simulink model "leg_contral_from_joy"  (R2024a)
settings: Solver=FixedStepDiscrete  StartTime=0.0  StopTime=inf  FixedStep=0.01  RelTol=1e-3  EnableMultiTasking=on
InitFcn:
  | run('robota_init.m')
values from neighbouring files (symbols this model uses):
  foot_step_x = single([0.647962241881123,0.669281948440417,0.689047458853030,0.707336632089232,0.724214871275340,0.739734081466605,0.753932398834638,0.766834545548556,0.778452679930586,0.788787625824203,0.797830378556315,0.805563797434742,0.811964406427908,0.817004235554845,0.820652645599333,0.822878088081130,0.823649760998204,0.822939128724922,0.820721281639968,0.816976117592065,0.811689333218330,0.804853218436 ...(+3308 chars)    [robota_init.m]
  foot_step_y = single([0.00431677655718721,0.0162618273816606,0.0344599539851875,0.0576998848000865,0.0849190036162384,0.115189239656799,0.147704049746776,0.181766425758056,0.216777863221598,0.252228229678260,0.287686473989677,0.322792120445942,0.357247494083859,0.390810626164481,0.423288791248474,0.454532629749211,0.484430812233581,0.512905204076631,0.539906491355785,0.565410231091200,0.589413291098898,0.611930 ...(+3410 chars)    [robota_init.m]
  height_plane = 0.025    [robota_init.m]
undefined symbols (not defined in the file or in its folder): axes, axes_SL_Info, buttons, buttons_SL_Info, foot_z, header, lb_alfa, lb_beta, lb_gamma, lf_alfa, lf_beta, lf_gamma, plane_x, plane_y, rb_alfa, rb_beta, rb_gamma, rf_alfa, rf_beta, rf_gamma, x, X, y, Y, z, Z
libraries: sm_lib x84, nesl_utility x21, hdlsllib x20, ros2lib x10, instrumentseriallib x2
(part 3 of 3)

== system leg_contral_from_joy/mutibody_sim/RB_Subsystem/L_jiont1 ==
  L_jiont : sm_lib/Body Elements/File Solid  ExtGeomFileName=STL/L_arm_joint.stl  UnitType=Custom  ExtGeomFileUnits=mm  StepReaderType=HEX  ExportConvexHullGeometry=off  InertiaType=Custom  BasedOnType=Density  Density=1000  DensityUnits=kg/m^3  Mass=100  MassUnits=g  CenterOfMass=[0 0 0]  CenterOfMassUnits=m  MomentsOfInertia=[1 1 1]  MomentsOfInertiaUnits=kg*m^2  ProductsOfInertia=[0 0 0]  ProductsOfInertiaUnits=kg*m^2  GraphicType=FromGeometry  MarkerShape=Sphere  MarkerSize=10  GraphicVisPropType=SimpleVisualProperties  GraphicDiffuseColor=[0.5 0.5 0.5]  GraphicOpacity=1.0  GraphicSpecularColor=[0.5 0.5 0.5 1.0]  GraphicAmbientColor=[0.15 0.15 0.15 1.0]  GraphicEmissiveColor=[0.0 0.0 0.0 1.0]  GraphicShininess=75  DoExposeReferenceFrame=on  SerializedFrames=<Frames/>
  L_jiont to Body : sm_lib/Frames and Transforms/Rigid Transform  RotationMethod=None  FollAlignAxisA=+Z  BaseAlignAxisA=+X  FollAlignAxisB=+Y  BaseAlignAxisB=+Z  RotationStandardAxis=+X  RotationAngle=180  RotationAngleUnits=deg  RotationArbitraryAxis=[0 0 1]  RotationSequenceAxes=FollowerAxes  RotationSequence=XYX  RotationSequenceAngles=[0 0 0]  RotationSequenceAnglesUnits=deg  RotationMatrix=[1 0 0; 0 1 0; 0 0 1]  Quaternion=[1 0 0 0]  TranslationMethod=Cartesian  TranslationCartesianOffset=[10 -13 9.5]  TranslationCartesianOffsetUnits=mm  TranslationStandardAxis=+Z  TranslationStandardOffset=100  TranslationStandardOffsetUnits=mm  TranslationROffset=0  TranslationROffsetUnits=m  TranslationThetaOffset=0  TranslationThetaOffsetUnits=deg  TranslationZOffset=0  TranslationZOffsetUnits=m
  L_jiont to Body1 : sm_lib/Frames and Transforms/Rigid Transform  RotationMethod=StandardAxis  FollAlignAxisA=+Z  BaseAlignAxisA=-Y  FollAlignAxisB=+Y  BaseAlignAxisB=+Z  RotationStandardAxis=+X  RotationAngle=90  RotationAngleUnits=deg  RotationArbitraryAxis=[0 0 1]  RotationSequenceAxes=FollowerAxes  RotationSequence=XYX  RotationSequenceAngles=[0 0 0]  RotationSequenceAnglesUnits=deg  RotationMatrix=[1 0 0; 0 1 0; 0 0 1]  Quaternion=[1 0 0 0]  TranslationMethod=None  TranslationCartesianOffset=[10 -13 0]  TranslationCartesianOffsetUnits=cm  TranslationStandardAxis=+Z  TranslationStandardOffset=100  TranslationStandardOffsetUnits=cm  TranslationROffset=0  TranslationROffsetUnits=m  TranslationThetaOffset=0  TranslationThetaOffsetUnits=deg  TranslationZOffset=0  TranslationZOffsetUnits=m
  "L_jiont to L_arm_ly " : sm_lib/Frames and Transforms/Rigid Transform  RotationMethod=AlignedAxes  FollAlignAxisA=+Z  BaseAlignAxisA=+X  FollAlignAxisB=+X  BaseAlignAxisB=+Y  RotationStandardAxis=+Y  RotationAngle=90  RotationAngleUnits=deg  RotationArbitraryAxis=[0 0 1]  RotationSequenceAxes=FollowerAxes  RotationSequence=XYX  RotationSequenceAngles=[0 0 0]  RotationSequenceAnglesUnits=deg  RotationMatrix=[1 0 0; 0 1 0; 0 0 1]  Quaternion=[1 0 0 0]  TranslationMethod=Cartesian  TranslationCartesianOffset=[37 10 20]  TranslationCartesianOffsetUnits=mm  TranslationStandardAxis=+Z  TranslationStandardOffset=100  TranslationStandardOffsetUnits=mm  TranslationROffset=0  TranslationROffsetUnits=m  TranslationThetaOffset=0  TranslationThetaOffsetUnits=deg  TranslationZOffset=0  TranslationZOffsetUnits=m
  L_jiont to L_arm_ly 1 : sm_lib/Frames and Transforms/Rigid Transform  RotationMethod=AlignedAxes  FollAlignAxisA=+Z  BaseAlignAxisA=-Z  FollAlignAxisB=+X  BaseAlignAxisB=-X  RotationStandardAxis=+Z  RotationAngle=180  RotationAngleUnits=deg  RotationArbitraryAxis=[0 0 1]  RotationSequenceAxes=FollowerAxes  RotationSequence=XYX  RotationSequenceAngles=[0 0 0]  RotationSequenceAnglesUnits=deg  RotationMatrix=[1 0 0; 0 1 0; 0 0 1]  Quaternion=[1 0 0 0]  TranslationMethod=None  TranslationCartesianOffset=[30 0 20]  TranslationCartesianOffsetUnits=cm  TranslationStandardAxis=+Z  TranslationStandardOffset=100  TranslationStandardOffsetUnits=cm  TranslationROffset=0  TranslationROffsetUnits=m  TranslationThetaOffset=0  TranslationThetaOffsetUnits=deg  TranslationZOffset=0  TranslationZOffsetUnits=m
  Conn1 : PMIOPort  Side=Left
  Conn2 : PMIOPort  Port=2  Side=Right
  connections:
  L_jiont to Body1/RConn1 -- Conn1/RConn1
  Conn2/RConn1 -- L_jiont to L_arm_ly 1/RConn1
  L_jiont to Body/LConn1 -- "L_jiont to L_arm_ly "/LConn1 -- L_jiont/RConn1
  L_jiont to L_arm_ly 1/LConn1 -- "L_jiont to L_arm_ly "/RConn1
  L_jiont to Body/RConn1 -- L_jiont to Body1/LConn1

== system leg_contral_from_joy/mutibody_sim/RB_Subsystem/R_arm Subsystem1 ==
  R_arm_ly : sm_lib/Body Elements/File Solid  ExtGeomFileName=STL/R_arm_ly.STL  UnitType=Custom  ExtGeomFileUnits=mm  StepReaderType=HEX  ExportConvexHullGeometry=off  InertiaType=Custom  BasedOnType=Mass  Density=1000  DensityUnits=kg/m^3  Mass=100  MassUnits=g  CenterOfMass=[10 0 -70]  CenterOfMassUnits=mm  MomentsOfInertia=[1 1 1]  MomentsOfInertiaUnits=kg*m^2  ProductsOfInertia=[0 0 0]  ProductsOfInertiaUnits=kg*m^2  GraphicType=FromGeometry  MarkerShape=Sphere  MarkerSize=10  GraphicVisPropType=SimpleVisualProperties  GraphicDiffuseColor=[0.5 0.5 0.5]  GraphicOpacity=1.0  GraphicSpecularColor=[0.5 0.5 0.5 1.0]  GraphicAmbientColor=[0.15 0.15 0.15 1.0]  GraphicEmissiveColor=[0.0 0.0 0.0 1.0]  GraphicShininess=75  DoExposeReferenceFrame=on  SerializedFrames=<Frames/>
  "R_arm_ly to R_wrist_ly " : sm_lib/Frames and Transforms/Rigid Transform  RotationMethod=AlignedAxes  FollAlignAxisA=-Z  BaseAlignAxisA=+Y  FollAlignAxisB=-Y  BaseAlignAxisB=+X  RotationStandardAxis=+X  RotationAngle=90  RotationAngleUnits=deg  RotationArbitraryAxis=[0 0 1]  RotationSequenceAxes=FollowerAxes  RotationSequence=XYX  RotationSequenceAngles=[0 0 0]  RotationSequenceAnglesUnits=deg  RotationMatrix=[1 0 0; 0 1 0; 0 0 1]  Quaternion=[1 0 0 0]  TranslationMethod=None  TranslationCartesianOffset=[-5 0 -8]  TranslationCartesianOffsetUnits=cm  TranslationStandardAxis=+Y  TranslationStandardOffset=40  TranslationStandardOffsetUnits=cm  TranslationROffset=0  TranslationROffsetUnits=m  TranslationThetaOffset=0  TranslationThetaOffsetUnits=deg  TranslationZOffset=0  TranslationZOffsetUnits=m
  R_arm_ly to R_wrist_ly 1 : sm_lib/Frames and Transforms/Rigid Transform  RotationMethod=StandardAxis  FollAlignAxisA=-Z  BaseAlignAxisA=+Y  FollAlignAxisB=-Y  BaseAlignAxisB=+X  RotationStandardAxis=+X  RotationAngle=180  RotationAngleUnits=deg  RotationArbitraryAxis=[0 0 1]  RotationSequenceAxes=FollowerAxes  RotationSequence=XYX  RotationSequenceAngles=[0 0 0]  RotationSequenceAnglesUnits=deg  RotationMatrix=[1 0 0; 0 1 0; 0 0 1]  Quaternion=[1 0 0 0]  TranslationMethod=None  TranslationCartesianOffset=[-5 0 -8]  TranslationCartesianOffsetUnits=cm  TranslationStandardAxis=+Y  TranslationStandardOffset=40  TranslationStandardOffsetUnits=cm  TranslationROffset=0  TranslationROffsetUnits=m  TranslationThetaOffset=0  TranslationThetaOffsetUnits=deg  TranslationZOffset=0  TranslationZOffsetUnits=m
  "R_arm_ly to R_jiont " : sm_lib/Frames and Transforms/Rigid Transform  RotationMethod=AlignedAxes  FollAlignAxisA=+Z  BaseAlignAxisA=+Y  FollAlignAxisB=+X  BaseAlignAxisB=+X  RotationStandardAxis=+X  RotationAngle=90  RotationAngleUnits=deg  RotationArbitraryAxis=[0 0 1]  RotationSequenceAxes=FollowerAxes  RotationSequence=XYX  RotationSequenceAngles=[0 0 0]  RotationSequenceAnglesUnits=deg  RotationMatrix=[1 0 0; 0 1 0; 0 0 1]  Quaternion=[1 0 0 0]  TranslationMethod=Cartesian  TranslationCartesianOffset=[14.5 12 -104.75]  TranslationCartesianOffsetUnits=mm  TranslationStandardAxis=+Z  TranslationStandardOffset=100  TranslationStandardOffsetUnits=mm  TranslationROffset=0  TranslationROffsetUnits=m  TranslationThetaOffset=0  TranslationThetaOffsetUnits=deg  TranslationZOffset=0  TranslationZOffsetUnits=m
  R_arm_ly to R_jiont1 : sm_lib/Frames and Transforms/Rigid Transform  RotationMethod=StandardAxis  FollAlignAxisA=+Z  BaseAlignAxisA=+X  FollAlignAxisB=+Y  BaseAlignAxisB=+Z  RotationStandardAxis=+Z  RotationAngle=180  RotationAngleUnits=deg  RotationArbitraryAxis=[0 0 1]  RotationSequenceAxes=FollowerAxes  RotationSequence=XYX  RotationSequenceAngles=[0 0 0]  RotationSequenceAnglesUnits=deg  RotationMatrix=[1 0 0; 0 1 0; 0 0 1]  Quaternion=[1 0 0 0]  TranslationMethod=None  TranslationCartesianOffset=[0 0 -50]  TranslationCartesianOffsetUnits=cm  TranslationStandardAxis=+Z  TranslationStandardOffset=100  TranslationStandardOffsetUnits=cm  TranslationROffset=0  TranslationROffsetUnits=m  TranslationThetaOffset=0  TranslationThetaOffsetUnits=deg  TranslationZOffset=0  TranslationZOffsetUnits=m
  Conn1 : PMIOPort  Side=Left
  Conn2 : PMIOPort  Port=2  Side=Right
  connections:
  R_arm_ly to R_wrist_ly 1/RConn1 -- Conn2/RConn1
  R_arm_ly to R_jiont1/LConn1 -- Conn1/RConn1
  "R_arm_ly to R_wrist_ly "/LConn1 -- R_arm_ly/RConn1 -- "R_arm_ly to R_jiont "/LConn1
  "R_arm_ly to R_wrist_ly "/RConn1 -- R_arm_ly to R_wrist_ly 1/LConn1
  R_arm_ly to R_jiont1/RConn1 -- "R_arm_ly to R_jiont "/RConn1

== system leg_contral_from_joy/mutibody_sim/RB_Subsystem/R_wrist Subsystem1 ==
  L_wrist_ly to foot : sm_lib/Frames and Transforms/Rigid Transform  RotationMethod=AlignedAxes  FollAlignAxisA=-Z  BaseAlignAxisA=+X  FollAlignAxisB=+X  BaseAlignAxisB=+Y  RotationStandardAxis=+X  RotationAngle=90  RotationAngleUnits=deg  RotationArbitraryAxis=[0 0 1]  RotationSequenceAxes=FollowerAxes  RotationSequence=XYX  RotationSequenceAngles=[0 0 0]  RotationSequenceAnglesUnits=deg  RotationMatrix=[1 0 0; 0 1 0; 0 0 1]  Quaternion=[1 0 0 0]  TranslationMethod=Cartesian  TranslationCartesianOffset=[116 0 0]  TranslationCartesianOffsetUnits=mm  TranslationStandardAxis=+Y  TranslationStandardOffset=40  TranslationStandardOffsetUnits=mm  TranslationROffset=0  TranslationROffsetUnits=m  TranslationThetaOffset=0  TranslationThetaOffsetUnits=deg  TranslationZOffset=0  TranslationZOffsetUnits=m
  R_wrist_ly : sm_lib/Body Elements/File Solid  ExtGeomFileName=STL/L_wrist_foot_ly.stl  UnitType=Custom  ExtGeomFileUnits=mm  StepReaderType=HEX  ExportConvexHullGeometry=off  InertiaType=Custom  BasedOnType=Density  Density=1000  DensityUnits=kg/m^3  Mass=100  MassUnits=g  CenterOfMass=[60 0 0]  CenterOfMassUnits=mm  MomentsOfInertia=[1 1 1]  MomentsOfInertiaUnits=kg*m^2  ProductsOfInertia=[0 0 0]  ProductsOfInertiaUnits=kg*m^2  GraphicType=FromGeometry  MarkerShape=Sphere  MarkerSize=10  GraphicVisPropType=SimpleVisualProperties  GraphicDiffuseColor=[0.5 0.5 0.5]  GraphicOpacity=1.0  GraphicSpecularColor=[0.5 0.5 0.5 1.0]  GraphicAmbientColor=[0.15 0.15 0.15 1.0]  GraphicEmissiveColor=[0.0 0.0 0.0 1.0]  GraphicShininess=75  DoExposeReferenceFrame=on  SerializedFrames=<Frames/>
  "R_wrist_ly to R_arm_ly " : sm_lib/Frames and Transforms/Rigid Transform  RotationMethod=StandardAxis  FollAlignAxisA=+Z  BaseAlignAxisA=+Y  FollAlignAxisB=+Y  BaseAlignAxisB=+Z  RotationStandardAxis=+X  RotationAngle=90  RotationAngleUnits=deg  RotationArbitraryAxis=[0 0 1]  RotationSequenceAxes=FollowerAxes  RotationSequence=XYX  RotationSequenceAngles=[0 0 0]  RotationSequenceAnglesUnits=deg  RotationMatrix=[1 0 0; 0 1 0; 0 0 1]  Quaternion=[1 0 0 0]  TranslationMethod=None  TranslationCartesianOffset=[-5 0 -8]  TranslationCartesianOffsetUnits=cm  TranslationStandardAxis=+Y  TranslationStandardOffset=40  TranslationStandardOffsetUnits=cm  TranslationROffset=0  TranslationROffsetUnits=m  TranslationThetaOffset=0  TranslationThetaOffsetUnits=deg  TranslationZOffset=0  TranslationZOffsetUnits=m
  Conn1 : PMIOPort  Side=Left
  Conn2 : PMIOPort  Port=2  Side=Right
  connections:
  Conn2/RConn1 -- L_wrist_ly to foot/RConn1
  Conn1/RConn1 -- "R_wrist_ly to R_arm_ly "/RConn1
  R_wrist_ly/RConn1 -- L_wrist_ly to foot/LConn1 -- "R_wrist_ly to R_arm_ly "/LConn1

== system leg_contral_from_joy/mutibody_sim/RF_Subsystem/R_arm Subsystem ==
  R_arm_ly : sm_lib/Body Elements/File Solid  ExtGeomFileName=STL/R_arm_ly.STL  UnitType=Custom  ExtGeomFileUnits=mm  StepReaderType=HEX  ExportConvexHullGeometry=off  InertiaType=Custom  BasedOnType=Mass  Density=1000  DensityUnits=kg/m^3  Mass=100  MassUnits=g  CenterOfMass=[10 0 -70]  CenterOfMassUnits=mm  MomentsOfInertia=[1 1 1]  MomentsOfInertiaUnits=kg*m^2  ProductsOfInertia=[0 0 0]  ProductsOfInertiaUnits=kg*m^2  GraphicType=FromGeometry  MarkerShape=Sphere  MarkerSize=10  GraphicVisPropType=SimpleVisualProperties  GraphicDiffuseColor=[0.5 0.5 0.5]  GraphicOpacity=1.0  GraphicSpecularColor=[0.5 0.5 0.5 1.0]  GraphicAmbientColor=[0.15 0.15 0.15 1.0]  GraphicEmissiveColor=[0.0 0.0 0.0 1.0]  GraphicShininess=75  DoExposeReferenceFrame=on  SerializedFrames=<Frames/>
  "R_arm_ly to R_wrist_ly " : sm_lib/Frames and Transforms/Rigid Transform  RotationMethod=AlignedAxes  FollAlignAxisA=-Z  BaseAlignAxisA=+Y  FollAlignAxisB=-Y  BaseAlignAxisB=+X  RotationStandardAxis=+X  RotationAngle=90  RotationAngleUnits=deg  RotationArbitraryAxis=[0 0 1]  RotationSequenceAxes=FollowerAxes  RotationSequence=XYX  RotationSequenceAngles=[0 0 0]  RotationSequenceAnglesUnits=deg  RotationMatrix=[1 0 0; 0 1 0; 0 0 1]  Quaternion=[1 0 0 0]  TranslationMethod=None  TranslationCartesianOffset=[-5 0 -8]  TranslationCartesianOffsetUnits=cm  TranslationStandardAxis=+Y  TranslationStandardOffset=40  TranslationStandardOffsetUnits=cm  TranslationROffset=0  TranslationROffsetUnits=m  TranslationThetaOffset=0  TranslationThetaOffsetUnits=deg  TranslationZOffset=0  TranslationZOffsetUnits=m
  R_arm_ly to R_wrist_ly 1 : sm_lib/Frames and Transforms/Rigid Transform  RotationMethod=StandardAxis  FollAlignAxisA=-Z  BaseAlignAxisA=+Y  FollAlignAxisB=-Y  BaseAlignAxisB=+X  RotationStandardAxis=+X  RotationAngle=180  RotationAngleUnits=deg  RotationArbitraryAxis=[0 0 1]  RotationSequenceAxes=FollowerAxes  RotationSequence=XYX  RotationSequenceAngles=[0 0 0]  RotationSequenceAnglesUnits=deg  RotationMatrix=[1 0 0; 0 1 0; 0 0 1]  Quaternion=[1 0 0 0]  TranslationMethod=None  TranslationCartesianOffset=[-5 0 -8]  TranslationCartesianOffsetUnits=cm  TranslationStandardAxis=+Y  TranslationStandardOffset=40  TranslationStandardOffsetUnits=cm  TranslationROffset=0  TranslationROffsetUnits=m  TranslationThetaOffset=0  TranslationThetaOffsetUnits=deg  TranslationZOffset=0  TranslationZOffsetUnits=m
  "R_arm_ly to R_jiont " : sm_lib/Frames and Transforms/Rigid Transform  RotationMethod=AlignedAxes  FollAlignAxisA=+Z  BaseAlignAxisA=+Y  FollAlignAxisB=+X  BaseAlignAxisB=+X  RotationStandardAxis=+X  RotationAngle=90  RotationAngleUnits=deg  RotationArbitraryAxis=[0 0 1]  RotationSequenceAxes=FollowerAxes  RotationSequence=XYX  RotationSequenceAngles=[0 0 0]  RotationSequenceAnglesUnits=deg  RotationMatrix=[1 0 0; 0 1 0; 0 0 1]  Quaternion=[1 0 0 0]  TranslationMethod=Cartesian  TranslationCartesianOffset=[14.5 12 -105.25]  TranslationCartesianOffsetUnits=mm  TranslationStandardAxis=+Z  TranslationStandardOffset=100  TranslationStandardOffsetUnits=mm  TranslationROffset=0  TranslationROffsetUnits=m  TranslationThetaOffset=0  TranslationThetaOffsetUnits=deg  TranslationZOffset=0  TranslationZOffsetUnits=m
  R_arm_ly to R_jiont1 : sm_lib/Frames and Transforms/Rigid Transform  RotationMethod=StandardAxis  FollAlignAxisA=+Z  BaseAlignAxisA=+X  FollAlignAxisB=+Y  BaseAlignAxisB=+Z  RotationStandardAxis=+Z  RotationAngle=180  RotationAngleUnits=deg  RotationArbitraryAxis=[0 0 1]  RotationSequenceAxes=FollowerAxes  RotationSequence=XYX  RotationSequenceAngles=[0 0 0]  RotationSequenceAnglesUnits=deg  RotationMatrix=[1 0 0; 0 1 0; 0 0 1]  Quaternion=[1 0 0 0]  TranslationMethod=None  TranslationCartesianOffset=[0 0 -50]  TranslationCartesianOffsetUnits=cm  TranslationStandardAxis=+Z  TranslationStandardOffset=100  TranslationStandardOffsetUnits=cm  TranslationROffset=0  TranslationROffsetUnits=m  TranslationThetaOffset=0  TranslationThetaOffsetUnits=deg  TranslationZOffset=0  TranslationZOffsetUnits=m
  Conn1 : PMIOPort  Side=Left
  Conn2 : PMIOPort  Port=2  Side=Right
  connections:
  R_arm_ly to R_jiont1/RConn1 -- "R_arm_ly to R_jiont "/RConn1
  "R_arm_ly to R_wrist_ly "/RConn1 -- R_arm_ly to R_wrist_ly 1/LConn1
  "R_arm_ly to R_jiont "/LConn1 -- R_arm_ly/RConn1 -- "R_arm_ly to R_wrist_ly "/LConn1
  R_arm_ly to R_jiont1/LConn1 -- Conn1/RConn1
  R_arm_ly to R_wrist_ly 1/RConn1 -- Conn2/RConn1

== system leg_contral_from_joy/mutibody_sim/RF_Subsystem/R_jiont Subsystem ==
  R_jiont : sm_lib/Body Elements/File Solid  ExtGeomFileName=STL/R_arm_joint_ly.stl  UnitType=Custom  ExtGeomFileUnits=mm  StepReaderType=HEX  ExportConvexHullGeometry=off  InertiaType=Custom  BasedOnType=Density  Density=1000  DensityUnits=kg/m^3  Mass=100  MassUnits=g  CenterOfMass=[0 0 0]  CenterOfMassUnits=m  MomentsOfInertia=[1 1 1]  MomentsOfInertiaUnits=kg*m^2  ProductsOfInertia=[0 0 0]  ProductsOfInertiaUnits=kg*m^2  GraphicType=FromGeometry  MarkerShape=Sphere  MarkerSize=10  GraphicVisPropType=SimpleVisualProperties  GraphicDiffuseColor=[0.5 0.5 0.5]  GraphicOpacity=1.0  GraphicSpecularColor=[0.5 0.5 0.5 1.0]  GraphicAmbientColor=[0.15 0.15 0.15 1.0]  GraphicEmissiveColor=[0.0 0.0 0.0 1.0]  GraphicShininess=75  DoExposeReferenceFrame=on  SerializedFrames=<Frames/>
  R_jiont to Body : sm_lib/Frames and Transforms/Rigid Transform  RotationMethod=None  FollAlignAxisA=+Z  BaseAlignAxisA=+X  FollAlignAxisB=+Y  BaseAlignAxisB=+Z  RotationStandardAxis=+X  RotationAngle=180  RotationAngleUnits=deg  RotationArbitraryAxis=[0 0 1]  RotationSequenceAxes=FollowerAxes  RotationSequence=XYX  RotationSequenceAngles=[0 0 0]  RotationSequenceAnglesUnits=deg  RotationMatrix=[1 0 0; 0 1 0; 0 0 1]  Quaternion=[1 0 0 0]  TranslationMethod=Cartesian  TranslationCartesianOffset=[17.5 -22 -10.2]  TranslationCartesianOffsetUnits=mm  TranslationStandardAxis=+Z  TranslationStandardOffset=100  TranslationStandardOffsetUnits=mm  TranslationROffset=0  TranslationROffsetUnits=m  TranslationThetaOffset=0  TranslationThetaOffsetUnits=deg  TranslationZOffset=0  TranslationZOffsetUnits=m
  R_jiont to Body1 : sm_lib/Frames and Transforms/Rigid Transform  RotationMethod=AlignedAxes  FollAlignAxisA=+Z  BaseAlignAxisA=-Y  FollAlignAxisB=-X  BaseAlignAxisB=-X  RotationStandardAxis=+X  RotationAngle=90  RotationAngleUnits=deg  RotationArbitraryAxis=[0 0 1]  RotationSequenceAxes=FollowerAxes  RotationSequence=XYX  RotationSequenceAngles=[0 0 0]  RotationSequenceAnglesUnits=deg  RotationMatrix=[1 0 0; 0 1 0; 0 0 1]  Quaternion=[1 0 0 0]  TranslationMethod=None  TranslationCartesianOffset=[10 -13 0]  TranslationCartesianOffsetUnits=cm  TranslationStandardAxis=+Z  TranslationStandardOffset=100  TranslationStandardOffsetUnits=cm  TranslationROffset=0  TranslationROffsetUnits=m  TranslationThetaOffset=0  TranslationThetaOffsetUnits=deg  TranslationZOffset=0  TranslationZOffsetUnits=m
  "R_jiont to R_arm_ly " : sm_lib/Frames and Transforms/Rigid Transform  RotationMethod=AlignedAxes  FollAlignAxisA=-Z  BaseAlignAxisA=+X  FollAlignAxisB=+X  BaseAlignAxisB=+Y  RotationStandardAxis=+Y  RotationAngle=90  RotationAngleUnits=deg  RotationArbitraryAxis=[0 0 1]  RotationSequenceAxes=FollowerAxes  RotationSequence=XYX  RotationSequenceAngles=[0 0 0]  RotationSequenceAnglesUnits=deg  RotationMatrix=[1 0 0; 0 1 0; 0 0 1]  Quaternion=[1 0 0 0]  TranslationMethod=Cartesian  TranslationCartesianOffset=[-10 1.5 0.5]  TranslationCartesianOffsetUnits=mm  TranslationStandardAxis=+Z  TranslationStandardOffset=100  TranslationStandardOffsetUnits=mm  TranslationROffset=0  TranslationROffsetUnits=m  TranslationThetaOffset=0  TranslationThetaOffsetUnits=deg  TranslationZOffset=0  TranslationZOffsetUnits=m
  R_jiont to R_arm_ly 1 : sm_lib/Frames and Transforms/Rigid Transform  RotationMethod=AlignedAxes  FollAlignAxisA=+Z  BaseAlignAxisA=-Z  FollAlignAxisB=+X  BaseAlignAxisB=+X  RotationStandardAxis=+Z  RotationAngle=0  RotationAngleUnits=deg  RotationArbitraryAxis=[0 0 1]  RotationSequenceAxes=FollowerAxes  RotationSequence=XYX  RotationSequenceAngles=[0 0 0]  RotationSequenceAnglesUnits=deg  RotationMatrix=[1 0 0; 0 1 0; 0 0 1]  Quaternion=[1 0 0 0]  TranslationMethod=None  TranslationCartesianOffset=[30 0 20]  TranslationCartesianOffsetUnits=cm  TranslationStandardAxis=+Z  TranslationStandardOffset=100  TranslationStandardOffsetUnits=cm  TranslationROffset=0  TranslationROffsetUnits=m  TranslationThetaOffset=0  TranslationThetaOffsetUnits=deg  TranslationZOffset=0  TranslationZOffsetUnits=m
  Conn1 : PMIOPort  Side=Left
  Conn2 : PMIOPort  Port=2  Side=Right
  connections:
  R_jiont/RConn1 -- R_jiont to Body/LConn1 -- "R_jiont to R_arm_ly "/LConn1
  R_jiont to Body1/RConn1 -- Conn1/RConn1
  R_jiont to R_arm_ly 1/LConn1 -- "R_jiont to R_arm_ly "/RConn1
  R_jiont to Body/RConn1 -- R_jiont to Body1/LConn1
  Conn2/RConn1 -- R_jiont to R_arm_ly 1/RConn1

== system leg_contral_from_joy/mutibody_sim/RF_Subsystem/R_wrist Subsystem ==
  L_wrist_ly to foot : sm_lib/Frames and Transforms/Rigid Transform  RotationMethod=AlignedAxes  FollAlignAxisA=-Z  BaseAlignAxisA=+X  FollAlignAxisB=+X  BaseAlignAxisB=+Y  RotationStandardAxis=+X  RotationAngle=90  RotationAngleUnits=deg  RotationArbitraryAxis=[0 0 1]  RotationSequenceAxes=FollowerAxes  RotationSequence=XYX  RotationSequenceAngles=[0 0 0]  RotationSequenceAnglesUnits=deg  RotationMatrix=[1 0 0; 0 1 0; 0 0 1]  Quaternion=[1 0 0 0]  TranslationMethod=Cartesian  TranslationCartesianOffset=[116 0 0]  TranslationCartesianOffsetUnits=mm  TranslationStandardAxis=+Y  TranslationStandardOffset=40  TranslationStandardOffsetUnits=mm  TranslationROffset=0  TranslationROffsetUnits=m  TranslationThetaOffset=0  TranslationThetaOffsetUnits=deg  TranslationZOffset=0  TranslationZOffsetUnits=m
  R_wrist_ly : sm_lib/Body Elements/File Solid  ExtGeomFileName=STL/L_wrist_foot_ly.stl  UnitType=Custom  ExtGeomFileUnits=mm  StepReaderType=HEX  ExportConvexHullGeometry=off  InertiaType=Custom  BasedOnType=Density  Density=1000  DensityUnits=kg/m^3  Mass=100  MassUnits=g  CenterOfMass=[60 0 0]  CenterOfMassUnits=mm  MomentsOfInertia=[1 1 1]  MomentsOfInertiaUnits=kg*m^2  ProductsOfInertia=[0 0 0]  ProductsOfInertiaUnits=kg*m^2  GraphicType=FromGeometry  MarkerShape=Sphere  MarkerSize=10  GraphicVisPropType=SimpleVisualProperties  GraphicDiffuseColor=[0.5 0.5 0.5]  GraphicOpacity=1.0  GraphicSpecularColor=[0.5 0.5 0.5 1.0]  GraphicAmbientColor=[0.15 0.15 0.15 1.0]  GraphicEmissiveColor=[0.0 0.0 0.0 1.0]  GraphicShininess=75  DoExposeReferenceFrame=on  SerializedFrames=<Frames/>
  "R_wrist_ly to R_arm_ly " : sm_lib/Frames and Transforms/Rigid Transform  RotationMethod=StandardAxis  FollAlignAxisA=+Z  BaseAlignAxisA=+Y  FollAlignAxisB=+Y  BaseAlignAxisB=+Z  RotationStandardAxis=+X  RotationAngle=90  RotationAngleUnits=deg  RotationArbitraryAxis=[0 0 1]  RotationSequenceAxes=FollowerAxes  RotationSequence=XYX  RotationSequenceAngles=[0 0 0]  RotationSequenceAnglesUnits=deg  RotationMatrix=[1 0 0; 0 1 0; 0 0 1]  Quaternion=[1 0 0 0]  TranslationMethod=None  TranslationCartesianOffset=[-5 0 -8]  TranslationCartesianOffsetUnits=cm  TranslationStandardAxis=+Y  TranslationStandardOffset=40  TranslationStandardOffsetUnits=cm  TranslationROffset=0  TranslationROffsetUnits=m  TranslationThetaOffset=0  TranslationThetaOffsetUnits=deg  TranslationZOffset=0  TranslationZOffsetUnits=m
  Conn1 : PMIOPort  Side=Left
  Conn2 : PMIOPort  Port=2  Side=Right
  connections:
  "R_wrist_ly to R_arm_ly "/LConn1 -- L_wrist_ly to foot/LConn1 -- R_wrist_ly/RConn1
  Conn1/RConn1 -- "R_wrist_ly to R_arm_ly "/RConn1
  Conn2/RConn1 -- L_wrist_ly to foot/RConn1

== matlab function leg_contral_from_joy/Joy_2_Leg_Angle/xyztoangle_rb ==
  data: alfa output; beta output; x input; gamma output; y input; z input
function [alfa,beta,gamma] = xyztoang(x,y,z)
%   此处显示详细说明

h  = 49.0;
hu = 125.5899;%sqrt(14.5^2+(104.75+20)^2)
hl = 116.0+20;

% y = h - y;

%UNTITLED 此处显示有关此函数的摘要
%   此处显示详细说明
% Some sqrt’s can be optimized out
dyz=sqrt(y.^2+z.^2);
lyz=sqrt(dyz.^2-h.^2);
gamma_yz=-atan(y./z);
gamma_h_offset=-atan(h./lyz);
gamma=gamma_yz-gamma_h_offset;
% #
lxzp=sqrt(lyz.^2+x.^2);
n=(lxzp.^2-hl^2-hu.^2)/(2*hu);
beta=-acos(n/hl);
% #
alfa_xzp=-atan(x/lyz);
alfa_off=acos((hu+n)/lxzp);
alfa=alfa_xzp+alfa_off;

== matlab function leg_contral_from_joy/Joy_2_Leg_Angle/MATLAB Function ==
  data: rpy_r input; rb_x output; rpy_p input; rpy_y input; pos_x input; pos_y input; pos_z input; rb_y output; rb_z output; rf_x output; rf_y output; rf_z output; lb_x output; lb_y output; lb_z output; lf_x output; lf_y output; lf_z output
function [rb_x,rb_y,rb_z, rf_x,rf_y,rf_z, lb_x,lb_y,lb_z, lf_x,lf_y,lf_z]  = pose_control(rpy_r,rpy_p,rpy_y,pos_x, pos_y, pos_z)
%UNTITLED3 此处显示有关此函数的摘要
%   此处显示详细说明
%   # 定义结构参数
  b = 78;%98;%78;%120;
  w = 10+98+78;%190;%120;
  l = 30;%250;
%   # 定义目标位姿
%   pos = np.mat([0.0,  0.0,  0.3 ]).T # 目标位置向量
%   rpy = np.array([0.0,  0.0,  0.0]) * math.pi / 180 # 欧拉角，化为弧度值
%   # 将欧拉角转换为旋转矩阵
%   R, P, Y = rpy[0], rpy[1], rpy[2]
    R = rpy_r;
    P = rpy_p;
    Y = rpy_y;
    pos = [pos_x, pos_y, pos_z]';
    rotx = ([[ 1,       0,       0     ]
             [ 0,       cos(R), -sin(R)]
             [ 0,       sin(R),  cos(R)]]);
    roty = ([[ cos(P),  0,      -sin(P)]
             [ 0,       1,       0     ]
             [ sin(P),  0,       cos(P)]]);
    rotz = ([[ cos(Y), -sin(Y),  0     ]
             [ sin(Y),  cos(Y),  0     ]
             [ 0,       0,       1     ]]);
  rot_mat = rotx * roty * rotz;
%   # 结构参数
    body_struc = ([[ l / 2,  b / 2,  0]     %rf
                   [ l / 2, -b / 2,  0]     %lf
                   [-l / 2,  b / 2,  0]     %rb
                   [-l / 2, -b / 2,  0]])'; %lb
    footpoint_struc = ([[ 0,  w / 2,  0]
                        [ 0, -w / 2,  0]
                        [ 0,  w / 2,  0]
                        [ 0, -w / 2,  0]])';
%     footpoint_struc = ([[ l / 2,  w / 2,  0]
%                         [ l / 2, -w / 2,  0]
%                         [-l / 2,  w / 2,  0]
%                         [-l / 2, -w / 2,  0]])';                    
                    
%     body_struc = ([[ l / 2,  b / 2,  0]     %rf
%                    [ l / 2, -b / 2,  0]     %lf
%                    [-l / 2,  b / 2,  0]     %rb
%                    [-l / 2, -b / 2,  0]])'; %lb
%     footpoint_struc = ([[ l / 2,  w / 2,  0]
%                         [ l / 2, -w / 2,  0]
%                         [-l / 2,  w / 2,  0]
%                         [-l / 2, -w / 2,  0]])';
%   # 计算单腿末端位置向量AB
  leg_pose = zeros(3, 4);
  for i = 1:4
%     leg_pose(:, i) = - pos - rot_mat * body_struc(:, i) + footpoint_struc(:, i);
    leg_pose(:, i) = pos + rot_mat * body_struc(:, i) - footpoint_struc(:, i);
  end
%     lf_x  = (leg_pose(1,1));
%     lf_y  = (leg_pose(2,1));
%     lf_z  = (leg_pose(3,1));
%     lb_x  = (leg_pose(1,2));
%     lb_y  = (leg_pose(2,2));
%     lb_z  = (leg_pose(3,2));
%     rf_x  = (leg_pose(1,3));
%     rf_y  = (leg_pose(2,3));
%     rf_z  = (leg_pose(3,3));
%     rb_x  = (leg_pose(1,4));
%     rb_y  = (leg_pose(2,4));
%     rb_z  = (leg_pose(3,4));

    rf_x  = (leg_pose(1,1));
    rf_y  = -(leg_pose(2,1));
    rf_z  = (leg_pose(3,1));
    lf_x  = (leg_pose(1,2));
    lf_y  = -(leg_pose(2,2));
    lf_z  = (leg_pose(3,2));
    rb_x  = (leg_pose(1,3));
    rb_y  = -(leg_pose(2,3));
    rb_z  = (leg_pose(3,3));
    lb_x  = (leg_pose(1,4));
    lb_y  = -(leg_pose(2,4));
    lb_z  = (leg_pose(3,4));
end

== matlab function leg_contral_from_joy/Joy_2_Leg_Angle/xyztoangle_rf ==
  data: alfa output; beta output; x input; gamma output; y input; z input
function [alfa,beta,gamma] = xyztoang(x,y,z)
%   此处显示详细说明

h  = 49.0;
hu = 125.5899;%sqrt(14.5^2+(104.75+20)^2)
hl = 116.0+20;

% y = h - y;

%UNTITLED 此处显示有关此函数的摘要
%   此处显示详细说明
% Some sqrt’s can be optimized out
dyz=sqrt(y.^2+z.^2);
lyz=sqrt(dyz.^2-h.^2);
gamma_yz=-atan(y./z);
gamma_h_offset=-atan(h./lyz);
gamma=gamma_yz-gamma_h_offset;
% #
lxzp=sqrt(lyz.^2+x.^2);
n=(lxzp.^2-hl^2-hu.^2)/(2*hu);
beta=-acos(n/hl);
% #
alfa_xzp=-atan(x/lyz);
alfa_off=acos((hu+n)/lxzp);
alfa=alfa_xzp+alfa_off;

== matlab function leg_contral_from_joy/Joy_2_Leg_Angle/xyztoangle_lb ==
  data: alfa output; beta output; x input; gamma output; y input; z input
function [alfa,beta,gamma] = xyztoang(x,y,z)
%   此处显示详细说明

h  = 49.0;
hu = 125.5899;%sqrt(14.5^2+(104.75+20)^2)
hl = 116.0+20;

% y = h - y;

%UNTITLED 此处显示有关此函数的摘要
%   此处显示详细说明
% Some sqrt’s can be optimized out
dyz=sqrt(y.^2+z.^2);
lyz=sqrt(dyz.^2-h.^2);
gamma_yz=-atan(y./z);
gamma_h_offset=-atan(h./lyz);
gamma=gamma_yz-gamma_h_offset;
% #
lxzp=sqrt(lyz.^2+x.^2);
n=(lxzp.^2-hl^2-hu.^2)/(2*hu);
beta=-acos(n/hl);
% #
alfa_xzp=-atan(x/lyz);
alfa_off=acos((hu+n)/lxzp);
alfa=alfa_xzp+alfa_off;

== matlab function leg_contral_from_joy/Joy_2_Leg_Angle/xyztoangle_lf ==
  data: alfa output; beta output; x input; gamma output; y input; z input
function [alfa,beta,gamma] = xyztoang(x,y,z)
%   此处显示详细说明

h  = 49.0;
hu = 125.5899;%sqrt(14.5^2+(104.75+20)^2)
hl = 116.0+20;

% y = h - y;

%UNTITLED 此处显示有关此函数的摘要
%   此处显示详细说明
% Some sqrt’s can be optimized out
dyz=sqrt(y.^2+z.^2);
lyz=sqrt(dyz.^2-h.^2);
gamma_yz=-atan(y./z);
gamma_h_offset=-atan(h./lyz);
gamma=gamma_yz-gamma_h_offset;
% #
lxzp=sqrt(lyz.^2+x.^2);
n=(lxzp.^2-hl^2-hu.^2)/(2*hu);
beta=-acos(n/hl);
% #
alfa_xzp=-atan(x/lyz);
alfa_off=acos((hu+n)/lxzp);
alfa=alfa_xzp+alfa_off;
